simulink library "FoldingMechanisms"  (R2017a)
settings: Solver=VariableStepAuto  StartTime=0.0  StopTime=10.0  RelTol=1e-3
undefined symbols (not defined in the file or in its folder): X, Y, Z
libraries: sm_lib x70, FoldingMechanisms x62, nesl_utility x7
(part 3 of 4)

== system FoldingMechanisms/Vertices/5-Foldlines Vertices ==
  5-Foldlines : Subsystem  mask{angspec=zeros(5,1), angval=zeros(5,1)}
      mask prompts: angspec "Specify initial angles [nx1] (1/0)"; angval "Initial angles [nx1]"
      mask DialogControl DescTextVar Prompt: 5-Foldlines Vertex
      mask DialogControl Control2 Prompt: Here you can define initial values for foldlines, i.e. the configuration (valley/mountain fold or elbow up/elbow down or +1/-1). Thereby, you can define an angle and simulink will try to use that as the inital pose. Note, contradicting specification may lead to unexpected results. Please provide a vector with the size of the number of foldlines. First, provide an vector containing 0 or 1 to specifiy whether you want to use the initial value or not. Then, specify the initial angles.
      mask Display:
      | %This does not require changes,
      | %when the number of foldlines is changed.
      | n_myfoldlines=5;
      | 
      | FoldChars={'A','B','C','D','E','F','G','H','I','J','K','L','M','N'};
      | M=[0.5;0.5];
      | %Draw point in the middle
      | theta = 0 : 0.01 : 2*pi;
      | patch([M(1)+0.03*cos(theta)], [M(2)+0.03*sin(theta)], [0.8 0 0]);
      | %Draw n foldlines
      | 
      | gap=0.05;
      | chargap=0.06;
      | textboxcorrection=[0.03;-0.003];
      | R=0.35;
      | phi=linspace(90,90-360,n_myfoldlines+1);
      | for idx=1:n_myfoldlines
      |     cl=[0 0 0];
      |     %Print blue, if angspec is defined
      |     if angspec(idx)
      |        cl=[0 0 0.8];
      |     end
      |     %if actfoldlines(idx)
      |     %    cl=[0.8 0 0];
      |     %end
      |     startpos=M+gap*[cosd(phi(idx));sind(phi(idx))];
      |     endpos=startpos+R*[cosd(phi(idx));sind(phi(idx))];
      |     textposline=(startpos+endpos)/2;
      |     textpos1=textposline+chargap*[cosd(phi(idx)+90);sind(phi(idx)+90)]-textboxcorrection;
      |     textpos2=textposline+chargap*[cosd(phi(idx)-90);sind(phi(idx)-90)]-textboxcorrection;
      |     patch([startpos(1);endpos(1)],[startpos(2);endpos(2)],cl);
      |     text(textpos1(1),textpos1(2),[FoldChars{idx},'.',num2str(idx)]);
      |     if idx<n_myfoldlines
      |         text(textpos2(1),textpos2(2),[FoldChars{idx+1},'.',num2str(idx)]);
      |     else
      |         text(textpos2(1),textpos2(2),[FoldChars{1},'.',num2str(idx)]);
      |     end
      | end
  5-Foldlines-MotionInput : Subsystem  mask{angspec=zeros(5,1), angval=zeros(5,1), actdrive1=off, actdrive2=off, actdrive3=off, actdrive4=off, actdrive5=off}
      mask prompts: angspec "Specify initial angles [nx1] (1/0)"; angval "Initial angles [nx1]"; actdrive1 "Actuate Foldline1"; actdrive2 "Actuate Foldline2"; actdrive3 "Actuate Foldline3"; actdrive4 "Actuate Foldline4"; actdrive5 "Actuate Foldline5"
      mask init:
      | %Please provide number of foldlines here
      | n_myfoldlines=5;
      | 
      | n_actuation=0;
      | inputselector=ones(n_myfoldlines,1);
      | for idx=1:n_myfoldlines
      |     if eval(['actdrive',num2str(idx)])
      |         n_actuation=n_actuation+1;
      |         inputselector(idx)=n_actuation;
      |     end 
      | end
      mask TypeOptions actdrive1: Foldline1/actdrive
      mask TypeOptions actdrive2: Foldline2/actdrive
      mask TypeOptions actdrive3: Foldline3/actdrive
      mask TypeOptions actdrive4: Foldline4/actdrive
      mask TypeOptions actdrive5: Foldline5/actdrive
      mask DialogControl DescTextVar Prompt: 5-Foldlines Vertex with motion input
      mask DialogControl Control2 Prompt: Here you can define initial values for foldlines, i.e. the configuration (valley/mountain fold or elbow up/elbow down or +1/-1). Thereby, you can define an angle and simulink will try to use that as the inital pose. Note, contradicting specification may lead to unexpected results. Please provide a vector with the size of the number of foldlines. First, provide an vector containing 0 or 1 to specifiy whether you want to use the initial value or not. Then, specify the initial angles.
      mask Display:
      | %Please provide number of foldlines here
      | n_myfoldlines=5;
      | 
      | %This does not require changes
      | n_actuation=0;
      | FoldChars={'A','B','C','D','E','F','G','H','I','J','K','L','M','N'};
      | 
      | M=[0.5;0.5];
      | %Draw point in the middle
      | theta = 0 : 0.01 : 2*pi;
      | patch([M(1)+0.03*cos(theta)], [M(2)+0.03*sin(theta)], [0.8 0 0]);
      | %Draw n foldlines
      | 
      | gap=0.05;
      | chargap=0.06;
      | textboxcorrection=[0.03;-0.003];
      | R=0.35;
      | phi=linspace(90,90-360,n_myfoldlines+1);
      | for idx=1:n_myfoldlines
      |     cl=[0 0 0];
      |     if eval(['actdrive',num2str(idx)])
      |         cl=[0.8 0 0];
      |         n_actuation=n_actuation+1;
      |     end
      |     startpos=M+gap*[cosd(phi(idx));sind(phi(idx))];
      |     endpos=startpos+R*[cosd(phi(idx));sind(phi(idx))];
      |     textposline=(startpos+endpos)/2;
      |     textpos1=textposline+chargap*[cosd(phi(idx)+90);sind(phi(idx)+90)]-textboxcorrection;
      |     textpos2=textposline+chargap*[cosd(phi(idx)-90);sind(phi(idx)-90)]-textboxcorrection;
      |     patch([startpos(1);endpos(1)],[startpos(2);endpos(2)],cl);
      |     text(textpos1(1),textpos1(2),[FoldChars{idx},'.',num2str(idx)]);
      |     if idx<n_myfoldlines
      |         text(textpos2(1),textpos2(2),[FoldChars{idx+1},'.',num2str(idx)]);
      |     else
      |         text(textpos2(1),textpos2(2),[FoldChars{1},'.',num2str(idx)]);
      |     end
      | end
      | 
      | text(0.75,0.1,['F=',num2str(n_myfoldlines-3-n_actuation)]);

== system FoldingMechanisms/Vertices/6-Foldlines Vertices ==
  6-Foldlines : Subsystem  mask{angspec=zeros(6,1), angval=zeros(6,1)}
      mask prompts: angspec "Specify initial angles [nx1] (1/0)"; angval "Initial angles [nx1]"
      mask DialogControl DescTextVar Prompt: 6-Foldlines Vertex
      mask DialogControl Control2 Prompt: Here you can define initial values for foldlines, i.e. the configuration (valley/mountain fold or elbow up/elbow down or +1/-1). Thereby, you can define an angle and simulink will try to use that as the inital pose. Note, contradicting specification may lead to unexpected results. Please provide a vector with the size of the number of foldlines. First, provide an vector containing 0 or 1 to specifiy whether you want to use the initial value or not. Then, specify the initial angles.
      mask Display:
      | %This does not require changes,
      | %when the number of foldlines is changed.
      | n_myfoldlines=6;
      | 
      | FoldChars={'A','B','C','D','E','F','G','H','I','J','K','L','M','N'};
      | M=[0.5;0.5];
      | %Draw point in the middle
      | theta = 0 : 0.01 : 2*pi;
      | patch([M(1)+0.03*cos(theta)], [M(2)+0.03*sin(theta)], [0.8 0 0]);
      | %Draw n foldlines
      | 
      | gap=0.05;
      | chargap=0.06;
      | textboxcorrection=[0.03;-0.003];
      | R=0.35;
      | phi=linspace(90,90-360,n_myfoldlines+1);
      | for idx=1:n_myfoldlines
      |     cl=[0 0 0];
      |     %Print blue, if angspec is defined
      |     if angspec(idx)
      |        cl=[0 0 0.8];
      |     end
      |     %if actfoldlines(idx)
      |     %    cl=[0.8 0 0];
      |     %end
      |     startpos=M+gap*[cosd(phi(idx));sind(phi(idx))];
      |     endpos=startpos+R*[cosd(phi(idx));sind(phi(idx))];
      |     textposline=(startpos+endpos)/2;
      |     textpos1=textposline+chargap*[cosd(phi(idx)+90);sind(phi(idx)+90)]-textboxcorrection;
      |     textpos2=textposline+chargap*[cosd(phi(idx)-90);sind(phi(idx)-90)]-textboxcorrection;
      |     patch([startpos(1);endpos(1)],[startpos(2);endpos(2)],cl);
      |     text(textpos1(1),textpos1(2),[FoldChars{idx},'.',num2str(idx)]);
      |     if idx<n_myfoldlines
      |         text(textpos2(1),textpos2(2),[FoldChars{idx+1},'.',num2str(idx)]);
      |     else
      |         text(textpos2(1),textpos2(2),[FoldChars{1},'.',num2str(idx)]);
      |     end
      | end
  6-Foldlines-MotionInput : Subsystem  mask{angspec=zeros(6,1), angval=zeros(6,1), actdrive1=off, actdrive2=off, actdrive3=off, actdrive4=off, actdrive5=off, actdrive6=off}
      mask prompts: angspec "Specify initial angles [nx1] (1/0)"; angval "Initial angles [nx1]"; actdrive1 "Actuate Foldline1"; actdrive2 "Actuate Foldline2"; actdrive3 "Actuate Foldline3"; actdrive4 "Actuate Foldline4"; actdrive5 "Actuate Foldline5"; actdrive6 "Actuate Foldline6"
      mask init:
      | %Please provide number of foldlines here
      | n_myfoldlines=6;
      | 
      | n_actuation=0;
      | inputselector=ones(n_myfoldlines,1);
      | for idx=1:n_myfoldlines
      |      %Force run of initization commands
      |     eval(['actdrive',num2str(idx),'=~actdrive',num2str(idx),';']);
      |     eval(['actdrive',num2str(idx),'=~actdrive',num2str(idx),';']);
      |     if eval(['actdrive',num2str(idx)])
      |         n_actuation=n_actuation+1;
      |         inputselector(idx)=n_actuation;
      |     end 
      | end
      mask TypeOptions actdrive1: Foldline1/actdrive
      mask TypeOptions actdrive2: Foldline2/actdrive
      mask TypeOptions actdrive3: Foldline3/actdrive
      mask TypeOptions actdrive4: Foldline4/actdrive
      mask TypeOptions actdrive5: Foldline5/actdrive
      mask TypeOptions actdrive6: Foldline6/actdrive
      mask DialogControl DescTextVar Prompt: 6-Foldlines Vertex with motion input
      mask DialogControl Control2 Prompt: Here you can define initial values for foldlines, i.e. the configuration (valley/mountain fold or elbow up/elbow down or +1/-1). Thereby, you can define an angle and simulink will try to use that as the inital pose. Note, contradicting specification may lead to unexpected results. Please provide a vector with the size of the number of foldlines. First, provide an vector containing 0 or 1 to specifiy whether you want to use the initial value or not. Then, specify the initial angles.
      mask Display:
      | %Please provide number of foldlines here
      | n_myfoldlines=6;
      | 
      | %This does not require changes
      | n_actuation=0;
      | FoldChars={'A','B','C','D','E','F','G','H','I','J','K','L','M','N'};
      | 
      | M=[0.5;0.5];
      | %Draw point in the middle
      | theta = 0 : 0.01 : 2*pi;
      | patch([M(1)+0.03*cos(theta)], [M(2)+0.03*sin(theta)], [0.8 0 0]);
      | %Draw n foldlines
      | 
      | gap=0.05;
      | chargap=0.06;
      | textboxcorrection=[0.03;-0.003];
      | R=0.35;
      | phi=linspace(90,90-360,n_myfoldlines+1);
      | for idx=1:n_myfoldlines
      |     cl=[0 0 0];
      |     if eval(['actdrive',num2str(idx)])
      |         cl=[0.8 0 0];
      |         n_actuation=n_actuation+1;
      |     end
      |     startpos=M+gap*[cosd(phi(idx));sind(phi(idx))];
      |     endpos=startpos+R*[cosd(phi(idx));sind(phi(idx))];
      |     textposline=(startpos+endpos)/2;
      |     textpos1=textposline+chargap*[cosd(phi(idx)+90);sind(phi(idx)+90)]-textboxcorrection;
      |     textpos2=textposline+chargap*[cosd(phi(idx)-90);sind(phi(idx)-90)]-textboxcorrection;
      |     patch([startpos(1);endpos(1)],[startpos(2);endpos(2)],cl);
      |     text(textpos1(1),textpos1(2),[FoldChars{idx},'.',num2str(idx)]);
      |     if idx<n_myfoldlines
      |         text(textpos2(1),textpos2(2),[FoldChars{idx+1},'.',num2str(idx)]);
      |     else
      |         text(textpos2(1),textpos2(2),[FoldChars{1},'.',num2str(idx)]);
      |     end
      | end
      | 
      | text(0.75,0.1,['F=',num2str(n_myfoldlines-3-n_actuation)]);

== system FoldingMechanisms/Vertices/7-Foldlines Vertices ==
  7-Foldlines : Subsystem  mask{angspec=zeros(7,1), angval=zeros(7,1)}
      mask prompts: angspec "Specify initial angles [nx1] (1/0)"; angval "Initial angles [nx1]"
      mask DialogControl DescTextVar Prompt: 7-Foldlines Vertex
      mask DialogControl Control2 Prompt: Here you can define initial values for foldlines, i.e. the configuration (valley/mountain fold or elbow up/elbow down or +1/-1). Thereby, you can define an angle and simulink will try to use that as the inital pose. Note, contradicting specification may lead to unexpected results. Please provide a vector with the size of the number of foldlines. First, provide an vector containing 0 or 1 to specifiy whether you want to use the initial value or not. Then, specify the initial angles.
      mask Display:
      | %This does not require changes,
      | %when the number of foldlines is changed.
      | n_myfoldlines=7;
      | 
      | FoldChars={'A','B','C','D','E','F','G','H','I','J','K','L','M','N'};
      | M=[0.5;0.5];
      | %Draw point in the middle
      | theta = 0 : 0.01 : 2*pi;
      | patch([M(1)+0.03*cos(theta)], [M(2)+0.03*sin(theta)], [0.8 0 0]);
      | %Draw n foldlines
      | 
      | gap=0.05;
      | chargap=0.06;
      | textboxcorrection=[0.03;-0.003];
      | R=0.35;
      | phi=linspace(90,90-360,n_myfoldlines+1);
      | for idx=1:n_myfoldlines
      |     cl=[0 0 0];
      |     %Print blue, if angspec is defined
      |     if angspec(idx)
      |        cl=[0 0 0.8];
      |     end
      |     %if actfoldlines(idx)
      |     %    cl=[0.8 0 0];
      |     %end
      |      startpos=M+gap*[cosd(phi(idx));sind(phi(idx))];
      |     endpos=startpos+R*[cosd(phi(idx));sind(phi(idx))];
      |     textposline=startpos+R/1.3*[cosd(phi(idx));sind(phi(idx))];
      |     textpos1=textposline+chargap*[cosd(phi(idx)+90);sind(phi(idx)+90)]-textboxcorrection;
      |     textpos2=textposline+chargap*[cosd(phi(idx)-90);sind(phi(idx)-90)]-textboxcorrection;
      |     patch([startpos(1);endpos(1)],[startpos(2);endpos(2)],cl);
      |     text(textpos1(1),textpos1(2),[FoldChars{idx},'.',num2str(idx)]);
      |     if idx<n_myfoldlines
      |         text(textpos2(1),textpos2(2),[FoldChars{idx+1},'.',num2str(idx)]);
      |     else
      |         text(textpos2(1),textpos2(2),[FoldChars{1},'.',num2str(idx)]);
      |     end
      | end
  7-Foldlines-MotionInput : Subsystem  mask{angspec=zeros(7,1), angval=zeros(7,1), actdrive1=off, actdrive2=off, actdrive3=off, actdrive4=off, actdrive5=off, actdrive6=off, actdrive7=off}
      mask prompts: angspec "Specify initial angles [nx1] (1/0)"; angval "Initial angles [nx1]"; actdrive1 "Actuate Foldline1"; actdrive2 "Actuate Foldline2"; actdrive3 "Actuate Foldline3"; actdrive4 "Actuate Foldline4"; actdrive5 "Actuate Foldline5"; actdrive6 "Actuate Foldline6"; actdrive7 "Actuate Foldline7"
      mask init:
      | %Please provide number of foldlines here
      | n_myfoldlines=7;
      | 
      | n_actuation=0;
      | inputselector=ones(n_myfoldlines,1);
      | for idx=1:n_myfoldlines
      |      %Force run of initization commands
      |     eval(['actdrive',num2str(idx),'=~actdrive',num2str(idx),';']);
      |     eval(['actdrive',num2str(idx),'=~actdrive',num2str(idx),';']);
      |     if eval(['actdrive',num2str(idx)])
      |         n_actuation=n_actuation+1;
      |         inputselector(idx)=n_actuation;
      |     end 
      | end
      mask TypeOptions actdrive1: Foldline1/actdrive
      mask TypeOptions actdrive2: Foldline2/actdrive
      mask TypeOptions actdrive3: Foldline3/actdrive
      mask TypeOptions actdrive4: Foldline4/actdrive
      mask TypeOptions actdrive5: Foldline5/actdrive
      mask TypeOptions actdrive6: Foldline6/actdrive
      mask TypeOptions actdrive7: Foldline7/actdrive
      mask DialogControl DescTextVar Prompt: 7-Foldlines Vertex with motion input
      mask DialogControl Control2 Prompt: Here you can define initial values for foldlines, i.e. the configuration (valley/mountain fold or elbow up/elbow down or +1/-1). Thereby, you can define an angle and simulink will try to use that as the inital pose. Note, contradicting specification may lead to unexpected results. Please provide a vector with the size of the number of foldlines. First, provide an vector containing 0 or 1 to specifiy whether you want to use the initial value or not. Then, specify the initial angles.
      mask Display:
      | %Please provide number of foldlines here
      | n_myfoldlines=7;
      | 
      | %This does not require changes
      | n_actuation=0;
      | FoldChars={'A','B','C','D','E','F','G','H','I','J','K','L','M','N'};
      | 
      | M=[0.5;0.5];
      | %Draw point in the middle
      | theta = 0 : 0.01 : 2*pi;
      | patch([M(1)+0.03*cos(theta)], [M(2)+0.03*sin(theta)], [0.8 0 0]);
      | %Draw n foldlines
      | 
      | gap=0.05;
      | chargap=0.06;
      | textboxcorrection=[0.03;-0.003];
      | R=0.35;
      | phi=linspace(90,90-360,n_myfoldlines+1);
      | for idx=1:n_myfoldlines
      |     cl=[0 0 0];
      |     if eval(['actdrive',num2str(idx)])
      |         cl=[0.8 0 0];
      |         n_actuation=n_actuation+1;
      |     end
      |     startpos=M+gap*[cosd(phi(idx));sind(phi(idx))];
      |     endpos=startpos+R*[cosd(phi(idx));sind(phi(idx))];
      |     textposline=startpos+R/1.3*[cosd(phi(idx));sind(phi(idx))];
      |     textpos1=textposline+chargap*[cosd(phi(idx)+90);sind(phi(idx)+90)]-textboxcorrection;
      |     textpos2=textposline+chargap*[cosd(phi(idx)-90);sind(phi(idx)-90)]-textboxcorrection;
      |     patch([startpos(1);endpos(1)],[startpos(2);endpos(2)],cl);
      |     text(textpos1(1),textpos1(2),[FoldChars{idx},'.',num2str(idx)]);
      |     if idx<n_myfoldlines
      |         text(textpos2(1),textpos2(2),[FoldChars{idx+1},'.',num2str(idx)]);
      |     else
      |         text(textpos2(1),textpos2(2),[FoldChars{1},'.',num2str(idx)]);
      |     end
      | end
      | 
      | text(0.75,0.1,['F=',num2str(n_myfoldlines-3-n_actuation)]);

== system FoldingMechanisms/Vertices/8-Foldlines Vertices ==
  8-Foldlines : Subsystem  mask{angspec=zeros(8,1), angval=zeros(8,1)}
      mask prompts: angspec "Specify initial angles [nx1] (1/0)"; angval "Initial angles [nx1]"
      mask DialogControl DescTextVar Prompt: 8-Foldlines Vertex
      mask DialogControl Control2 Prompt: Here you can define initial values for foldlines, i.e. the configuration (valley/mountain fold or elbow up/elbow down or +1/-1). Thereby, you can define an angle and simulink will try to use that as the inital pose. Note, contradicting specification may lead to unexpected results. Please provide a vector with the size of the number of foldlines. First, provide an vector containing 0 or 1 to specifiy whether you want to use the initial value or not. Then, specify the initial angles.
      mask Display:
      | %This does not require changes,
      | %when the number of foldlines is changed.
      | n_myfoldlines=8;
      | 
      | FoldChars={'A','B','C','D','E','F','G','H','I','J','K','L','M','N'};
      | M=[0.5;0.5];
      | %Draw point in the middle
      | theta = 0 : 0.01 : 2*pi;
      | patch([M(1)+0.03*cos(theta)], [M(2)+0.03*sin(theta)], [0.8 0 0]);
      | %Draw n foldlines
      | 
      | gap=0.05;
      | chargap=0.06;
      | textboxcorrection=[0.03;-0.003];
      | R=0.35;
      | phi=linspace(90,90-360,n_myfoldlines+1);
      | for idx=1:n_myfoldlines
      |     cl=[0 0 0];
      |     %Print blue, if angspec is defined
      |     if angspec(idx)
      |        cl=[0 0 0.8];
      |     end
      |     %if actfoldlines(idx)
      |     %    cl=[0.8 0 0];
      |     %end
      |      startpos=M+gap*[cosd(phi(idx));sind(phi(idx))];
      |     endpos=startpos+R*[cosd(phi(idx));sind(phi(idx))];
      |     textposline=startpos+R/1.25*[cosd(phi(idx));sind(phi(idx))];
      |     textpos1=textposline+chargap*[cosd(phi(idx)+90);sind(phi(idx)+90)]-textboxcorrection;
      |     textpos2=textposline+chargap*[cosd(phi(idx)-90);sind(phi(idx)-90)]-textboxcorrection;
      |     patch([startpos(1);endpos(1)],[startpos(2);endpos(2)],cl);
      |     text(textpos1(1),textpos1(2),[FoldChars{idx},'.',num2str(idx)]);
      |     if idx<n_myfoldlines
      |         text(textpos2(1),textpos2(2),[FoldChars{idx+1},'.',num2str(idx)]);
      |     else
      |         text(textpos2(1),textpos2(2),[FoldChars{1},'.',num2str(idx)]);
      |     end
      | end
  8-Foldlines-MotionInput : Subsystem  mask{angspec=zeros(8,1), angval=zeros(8,1), actdrive1=off, actdrive2=off, actdrive3=off, actdrive4=off, actdrive5=off, actdrive6=off, actdrive7=off, actdrive8=off}
      mask prompts: angspec "Specify initial angles [nx1] (1/0)"; angval "Initial angles [nx1]"; actdrive1 "Actuate Foldline1"; actdrive2 "Actuate Foldline2"; actdrive3 "Actuate Foldline3"; actdrive4 "Actuate Foldline4"; actdrive5 "Actuate Foldline5"; actdrive6 "Actuate Foldline6"; actdrive7 "Actuate Foldline7"; actdrive8 "Actuate Foldline8"
      mask init:
      | %Please provide number of foldlines here
      | n_myfoldlines=8;
      | 
      | n_actuation=0;
      | inputselector=ones(n_myfoldlines,1);
      | for idx=1:n_myfoldlines
      |      %Force run of initization commands
      |     eval(['actdrive',num2str(idx),'=~actdrive',num2str(idx),';']);
      |     eval(['actdrive',num2str(idx),'=~actdrive',num2str(idx),';']);
      |     if eval(['actdrive',num2str(idx)])
      |         n_actuation=n_actuation+1;
      |         inputselector(idx)=n_actuation;
      |     end 
      | end
      mask TypeOptions actdrive1: Foldline1/actdrive
      mask TypeOptions actdrive2: Foldline2/actdrive
      mask TypeOptions actdrive3: Foldline3/actdrive
      mask TypeOptions actdrive4: Foldline4/actdrive
      mask TypeOptions actdrive5: Foldline5/actdrive
      mask TypeOptions actdrive6: Foldline6/actdrive
      mask TypeOptions actdrive7: Foldline7/actdrive
      mask TypeOptions actdrive8: Foldline8/actdrive
      mask DialogControl DescTextVar Prompt: 8-Foldlines Vertex with motion input
      mask DialogControl Control2 Prompt: Here you can define initial values for foldlines, i.e. the configuration (valley/mountain fold or elbow up/elbow down or +1/-1). Thereby, you can define an angle and simulink will try to use that as the inital pose. Note, contradicting specification may lead to unexpected results. Please provide a vector with the size of the number of foldlines. First, provide an vector containing 0 or 1 to specifiy whether you want to use the initial value or not. Then, specify the initial angles.
      mask Display:
      | %Please provide number of foldlines here
      | n_myfoldlines=8;
      | 
      | %This does not require changes
      | n_actuation=0;
      | FoldChars={'A','B','C','D','E','F','G','H','I','J','K','L','M','N'};
      | 
      | M=[0.5;0.5];
      | %Draw point in the middle
      | theta = 0 : 0.01 : 2*pi;
      | patch([M(1)+0.03*cos(theta)], [M(2)+0.03*sin(theta)], [0.8 0 0]);
      | %Draw n foldlines
      | 
      | gap=0.05;
      | chargap=0.06;
      | textboxcorrection=[0.03;-0.003];
      | R=0.35;
      | phi=linspace(90,90-360,n_myfoldlines+1);
      | for idx=1:n_myfoldlines
      |     cl=[0 0 0];
      |     if eval(['actdrive',num2str(idx)])
      |         cl=[0.8 0 0];
      |         n_actuation=n_actuation+1;
      |     end
      |     startpos=M+gap*[cosd(phi(idx));sind(phi(idx))];
      |     endpos=startpos+R*[cosd(phi(idx));sind(phi(idx))];
      |     textposline=startpos+R/1.3*[cosd(phi(idx));sind(phi(idx))];
      |     textpos1=textposline+chargap*[cosd(phi(idx)+90);sind(phi(idx)+90)]-textboxcorrection;
      |     textpos2=textposline+chargap*[cosd(phi(idx)-90);sind(phi(idx)-90)]-textboxcorrection;
      |     patch([startpos(1);endpos(1)],[startpos(2);endpos(2)],cl);
      |     text(textpos1(1),textpos1(2),[FoldChars{idx},'.',num2str(idx)]);
      |     if idx<n_myfoldlines
      |         text(textpos2(1),textpos2(2),[FoldChars{idx+1},'.',num2str(idx)]);
      |     else
      |         text(textpos2(1),textpos2(2),[FoldChars{1},'.',num2str(idx)]);
      |     end
      | end
      | 
      | text(0.75,0.1,['F=',num2str(n_myfoldlines-3-n_actuation)]);

== system FoldingMechanisms/Vertices/Subelements ==
  Single Driven Foldline : Subsystem
      mask DialogControl DescGroupVar Prompt: Single Driven Foldline
      mask DialogControl DescTextVar Prompt: This block provides a single driven Foldline.
      mask Display: patch([0.5 0.5],[0.2 0.8],[0.8 0 0]);
  Single Foldline : Subsystem  mask{angleAB=0, specAngleAB=0}
      mask prompts: angleAB "Angle [°]"; specAngleAB "Specify Configuration [true/false]"
      mask init:
      | %Initialize
      | if (specAngleAB==true)
      |     set_param([gcb,'/Foldline'], 'PositionTargetSpecify','on');
      | else
      |     set_param([gcb,'/Foldline'], 'PositionTargetSpecify','off');
      | end
      mask DialogControl DescTextVar Prompt: This block provides the definition of a single Foldline with the possibility to specify the configuration
      mask Display: plot([0.5 0.5],[0.2 0.8]);
  Variant Foldline : Subsystem  LoadFcn=|  Variant=on  OverrideUsingVariant=Foldline  mask{angleAB=0, specAngleAB=0, actdrive=off, chooseVariant=Foldline}
      | actdrive = get_param(gcb,'actdrive');
      | if strcmp(actdrive,'on')
      |     set_param(gcb,'chooseVariant','Drive');
      | else
      |     set_param(gcb,'chooseVariant','Foldline');
      | end
      mask prompts: angleAB "Angle [°]"; specAngleAB "Specify Configuration [true/false]"; actdrive "Driven"; chooseVariant "Simulink:blkprm_prompts:OverrideUsingVariant"
      mask init:
      | actdrive = get_param(gcb,'actdrive');
      | if strcmp(actdrive,'on')
      |     set_param(gcb,'chooseVariant','Drive');
      | else
      |     set_param(gcb,'chooseVariant','Foldline');
      | end
      mask Callback actdrive:
      | actdrive = get_param(gcb,'actdrive');
      | if strcmp(actdrive,'on')
      |     set_param(gcb,'chooseVariant','Drive');
      | else
      |     set_param(gcb,'chooseVariant','Foldline');
      | end
      mask TypeOptions chooseVariant: OverrideUsingVariant
      mask DialogControl DescTextVar Prompt: This is a variant Foldline. You can choose, whether this Foldline is actuated. If actuated, Foldline specifications will be ignored. If not actuated, the drive function will be ignored.
      mask Display:
      | if strcmp(actdrive,'on');
      |     patch([0.5 0.5],[0.2 0.8],[0.8 0 0]);
      | else
      |     patch([0.5 0.5],[0.2 0.8],[0 0 0]);
      | end

== system FoldingMechanisms/Vertices/4-Foldlines Vertices/4-Foldlines ==
  Bus Creator4 : BusCreator  Inputs=4
  Foldline AB : FoldingMechanisms/Vertices/Subelements/Single Foldline  angleAB=angval(1)  specAngleAB=angspec(1)
      settings: SourceProductName=FoldingMechanisms
  Foldline AD : FoldingMechanisms/Vertices/Subelements/Single Foldline  angleAB=angval(4)  specAngleAB=angspec(4)
      settings: SourceProductName=FoldingMechanisms
  Foldline CB : FoldingMechanisms/Vertices/Subelements/Single Foldline  angleAB=angval(2)  specAngleAB=angspec(2)
      settings: SourceProductName=FoldingMechanisms
  Foldline CD : FoldingMechanisms/Vertices/Subelements/Single Foldline  angleAB=angval(3)  specAngleAB=angspec(2)
      settings: SourceProductName=FoldingMechanisms
  A1 : PMIOPort  Port=1  Side=Left
  A4 : PMIOPort  Port=2  Side=Left
  D4 : PMIOPort  Port=3  Side=Left
  D3 : PMIOPort  Port=4  Side=Left
  B1 : PMIOPort  Port=5  Side=Right
  B2 : PMIOPort  Port=6  Side=Right
  C2 : PMIOPort  Port=7  Side=Right
  C3 : PMIOPort  Port=8  Side=Right
  Out Bus Element : Outport  PortName=OutBus  Element=Sensing
  wires:
  Bus Creator4/1 -> Out Bus Element/1
  Foldline AB/1 -> Bus Creator4/1
  Foldline AD/1 -> Bus Creator4/4
  Foldline CD/1 -> Bus Creator4/3
  Foldline CB/1 -> Bus Creator4/2
  connections:
  Foldline CB/RConn1 -- B2/RConn1
  Foldline AB/LConn1 -- A1/RConn1
  Foldline AB/RConn1 -- B1/RConn1
  D4/RConn1 -- Foldline AD/LConn1
  A4/RConn1 -- Foldline AD/RConn1
  Foldline CD/LConn1 -- D3/RConn1
  Foldline CD/RConn1 -- C3/RConn1
  C2/RConn1 -- Foldline CB/LConn1

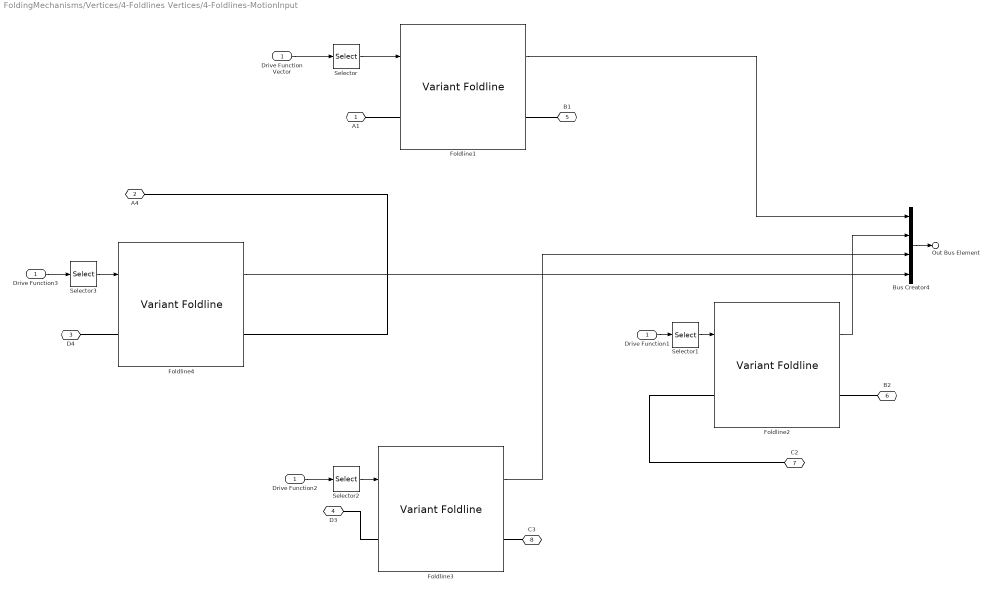
== system FoldingMechanisms/Vertices/4-Foldlines Vertices/4-Foldlines-MotionInput ==
  Drive Function Vector : Inport
  Bus Creator4 : BusCreator  Inputs=4
  Drive Function1 : InportShadow
  Drive Function2 : InportShadow
  Drive Function3 : InportShadow
  Foldline1 : FoldingMechanisms/Vertices/Subelements/Variant Foldline  angleAB=angval(1)  specAngleAB=angspec(1)  actdrive=off  chooseVariant=Foldline
      settings: SourceProductName=FoldingMechanisms
  Foldline2 : FoldingMechanisms/Vertices/Subelements/Variant Foldline  angleAB=angval(2)  specAngleAB=angspec(2)  actdrive=off  chooseVariant=Foldline
      settings: SourceProductName=FoldingMechanisms
  Foldline3 : FoldingMechanisms/Vertices/Subelements/Variant Foldline  angleAB=angval(3)  specAngleAB=angspec(3)  actdrive=off  chooseVariant=Foldline
      settings: SourceProductName=FoldingMechanisms
  Foldline4 : FoldingMechanisms/Vertices/Subelements/Variant Foldline  angleAB=angval(4)  specAngleAB=angspec(4)  actdrive=off  chooseVariant=Foldline
      settings: SourceProductName=FoldingMechanisms
  Selector : Selector  InputPortWidth=max(n_actuation,1)  IndexOptions=Index vector (dialog)  Indices=inputselector(1)  OutputSizes=1
  Selector1 : Selector  InputPortWidth=max(n_actuation,1)  IndexOptions=Index vector (dialog)  Indices=inputselector(2)  OutputSizes=1
  Selector2 : Selector  InputPortWidth=max(n_actuation,1)  IndexOptions=Index vector (dialog)  Indices=inputselector(3)  OutputSizes=1
  Selector3 : Selector  InputPortWidth=max(n_actuation,1)  IndexOptions=Index vector (dialog)  Indices=inputselector(4)  OutputSizes=1
  A1 : PMIOPort  Port=1  Side=Left
  A4 : PMIOPort  Port=2  Side=Left
  D4 : PMIOPort  Port=3  Side=Left
  D3 : PMIOPort  Port=4  Side=Left
  B1 : PMIOPort  Port=5  Side=Right
  B2 : PMIOPort  Port=6  Side=Right
  C2 : PMIOPort  Port=7  Side=Right
  C3 : PMIOPort  Port=8  Side=Right
  Out Bus Element : Outport  PortName=OutBus  Element=Sensing
  wires:
  Bus Creator4/1 -> Out Bus Element/1
  Drive Function Vector/1 -> Selector/1
  Foldline1/1 -> Bus Creator4/1
  Foldline4/1 -> Bus Creator4/4
  Foldline3/1 -> Bus Creator4/3
  Foldline2/1 -> Bus Creator4/2
  Drive Function1/1 -> Selector1/1
  Drive Function2/1 -> Selector2/1
  Drive Function3/1 -> Selector3/1
  Selector/1 -> Foldline1/1
  Selector1/1 -> Foldline2/1
  Selector2/1 -> Foldline3/1
  Selector3/1 -> Foldline4/1
  connections:
  Foldline2/RConn1 -- B2/RConn1
  Foldline1/LConn1 -- A1/RConn1
  Foldline1/RConn1 -- B1/RConn1
  Foldline4/LConn1 -- D4/RConn1
  Foldline4/RConn1 -- A4/RConn1
  Foldline3/LConn1 -- D3/RConn1
  Foldline3/RConn1 -- C3/RConn1
  Foldline2/LConn1 -- C2/RConn1

== system FoldingMechanisms/Vertices/5-Foldlines Vertices/5-Foldlines ==
  Bus Creator4 : BusCreator  Inputs=5
  Foldline AB : FoldingMechanisms/Vertices/Subelements/Single Foldline  angleAB=angval(1)  specAngleAB=angspec(1)
      settings: SourceProductName=FoldingMechanisms
  Foldline AD : FoldingMechanisms/Vertices/Subelements/Single Foldline  angleAB=angval(4)  specAngleAB=angspec(4)
      settings: SourceProductName=FoldingMechanisms
  Foldline AD1 : FoldingMechanisms/Vertices/Subelements/Single Foldline  angleAB=angval(4)  specAngleAB=angspec(4)
      settings: SourceProductName=FoldingMechanisms
  Foldline CB : FoldingMechanisms/Vertices/Subelements/Single Foldline  angleAB=angval(2)  specAngleAB=angspec(2)
      settings: SourceProductName=FoldingMechanisms
  Foldline CD : FoldingMechanisms/Vertices/Subelements/Single Foldline  angleAB=angval(3)  specAngleAB=angspec(2)
      settings: SourceProductName=FoldingMechanisms
  A1 : PMIOPort  Port=1  Side=Left
  A5 : PMIOPort  Port=2  Side=Left
  E5 : PMIOPort  Port=3  Side=Left
  E4 : PMIOPort  Port=4  Side=Left
  D4 : PMIOPort  Port=5  Side=Left
  B1 : PMIOPort  Port=6  Side=Right
  B2 : PMIOPort  Port=7  Side=Right
  C2 : PMIOPort  Port=8  Side=Right
  C3 : PMIOPort  Port=9  Side=Right
  D3 : PMIOPort  Port=10  Side=Right
  Out Bus Element : Outport  PortName=OutBus  Element=Sensing
  wires:
  Bus Creator4/1 -> Out Bus Element/1
  Foldline AB/1 -> Bus Creator4/1
  Foldline AD/1 -> Bus Creator4/4
  Foldline CD/1 -> Bus Creator4/3
  Foldline CB/1 -> Bus Creator4/2
  Foldline AD1/1 -> Bus Creator4/5
  connections:
  Foldline CB/RConn1 -- B2/RConn1
  Foldline AB/LConn1 -- A1/RConn1
  Foldline AB/RConn1 -- B1/RConn1
  D4/RConn1 -- Foldline AD/LConn1
  E4/RConn1 -- Foldline AD/RConn1
  Foldline CD/LConn1 -- D3/RConn1
  Foldline CD/RConn1 -- C3/RConn1
  C2/RConn1 -- Foldline CB/LConn1
  A5/RConn1 -- Foldline AD1/RConn1
  E5/RConn1 -- Foldline AD1/LConn1

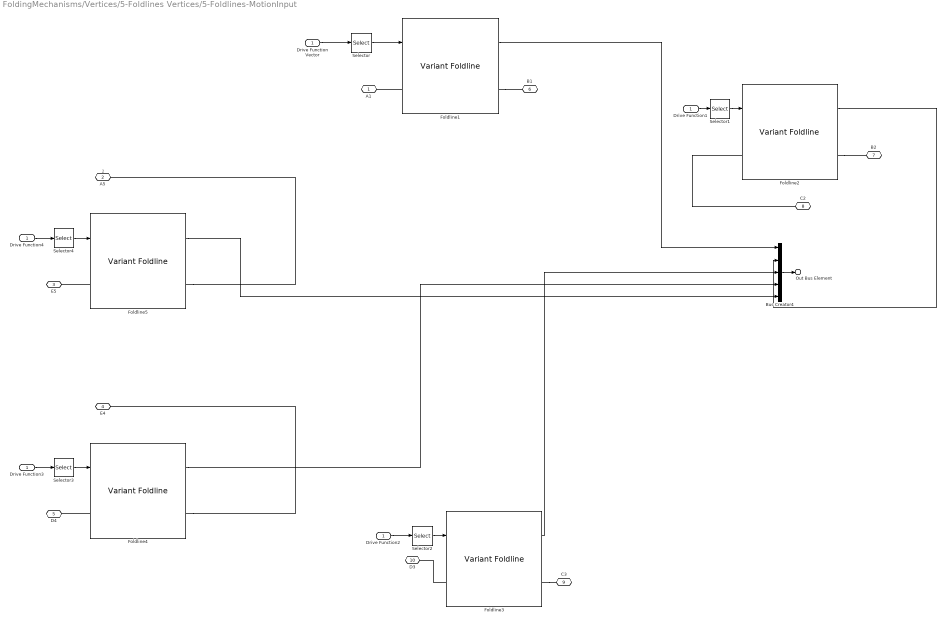
== system FoldingMechanisms/Vertices/5-Foldlines Vertices/5-Foldlines-MotionInput ==
  note: 2
  Drive Function Vector : Inport
  Bus Creator4 : BusCreator  Inputs=5
  Drive Function{1..4} (4 alike) : InportShadow
  Foldline1 : FoldingMechanisms/Vertices/Subelements/Variant Foldline  angleAB=angval(1)  specAngleAB=angspec(1)  actdrive=off  chooseVariant=Foldline
      settings: SourceProductName=FoldingMechanisms
  Foldline2 : FoldingMechanisms/Vertices/Subelements/Variant Foldline  angleAB=angval(2)  specAngleAB=angspec(2)  actdrive=off  chooseVariant=Foldline
      settings: SourceProductName=FoldingMechanisms
  Foldline3 : FoldingMechanisms/Vertices/Subelements/Variant Foldline  angleAB=angval(3)  specAngleAB=angspec(3)  actdrive=off  chooseVariant=Foldline
      settings: SourceProductName=FoldingMechanisms
  Foldline4 : FoldingMechanisms/Vertices/Subelements/Variant Foldline  angleAB=angval(4)  specAngleAB=angspec(4)  actdrive=off  chooseVariant=Foldline
      settings: SourceProductName=FoldingMechanisms
  Foldline5 : FoldingMechanisms/Vertices/Subelements/Variant Foldline  angleAB=angval(5)  specAngleAB=angspec(5)  actdrive=off  chooseVariant=Foldline
      settings: SourceProductName=FoldingMechanisms
  Selector : Selector  InputPortWidth=max(n_actuation,1)  IndexOptions=Index vector (dialog)  Indices=inputselector(1)  OutputSizes=1
  Selector1 : Selector  InputPortWidth=max(n_actuation,1)  IndexOptions=Index vector (dialog)  Indices=inputselector(2)  OutputSizes=1
  Selector2 : Selector  InputPortWidth=max(n_actuation,1)  IndexOptions=Index vector (dialog)  Indices=inputselector(3)  OutputSizes=1
  Selector3 : Selector  InputPortWidth=max(n_actuation,1)  IndexOptions=Index vector (dialog)  Indices=inputselector(4)  OutputSizes=1
  Selector4 : Selector  InputPortWidth=max(n_actuation,1)  IndexOptions=Index vector (dialog)  Indices=inputselector(5)  OutputSizes=1
  A1 : PMIOPort  Port=1  Side=Left
  A5 : PMIOPort  Port=2  Side=Left
  E5 : PMIOPort  Port=3  Side=Left
  E4 : PMIOPort  Port=4  Side=Left
  D4 : PMIOPort  Port=5  Side=Left
  B1 : PMIOPort  Port=6  Side=Right
  B2 : PMIOPort  Port=7  Side=Right
  C2 : PMIOPort  Port=8  Side=Right
  C3 : PMIOPort  Port=9  Side=Right
  D3 : PMIOPort  Port=10  Side=Right
  Out Bus Element : Outport  PortName=OutBus  Element=Sensing
  wires:
  Bus Creator4/1 -> Out Bus Element/1
  Drive Function Vector/1 -> Selector/1
  Foldline1/1 -> Bus Creator4/1
  Foldline4/1 -> Bus Creator4/4
  Foldline3/1 -> Bus Creator4/3
  Foldline2/1 -> Bus Creator4/2
  Drive Function1/1 -> Selector1/1
  Drive Function2/1 -> Selector2/1
  Drive Function3/1 -> Selector3/1
  Selector/1 -> Foldline1/1
  Selector1/1 -> Foldline2/1
  Selector2/1 -> Foldline3/1
  Selector3/1 -> Foldline4/1
  Drive Function4/1 -> Selector4/1
  Selector4/1 -> Foldline5/1
  Foldline5/1 -> Bus Creator4/5
  connections:
  Foldline2/RConn1 -- B2/RConn1
  Foldline1/LConn1 -- A1/RConn1
  Foldline1/RConn1 -- B1/RConn1
  Foldline4/LConn1 -- D4/RConn1
  Foldline4/RConn1 -- E4/RConn1
  Foldline3/LConn1 -- D3/RConn1
  Foldline3/RConn1 -- C3/RConn1
  Foldline2/LConn1 -- C2/RConn1
  Foldline5/LConn1 -- E5/RConn1
  Foldline5/RConn1 -- A5/RConn1

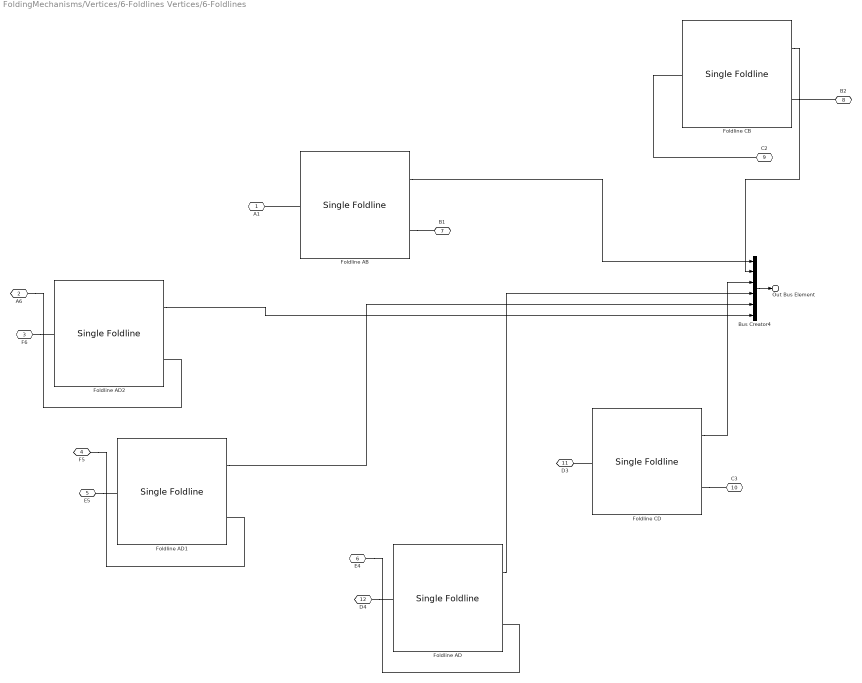
== system FoldingMechanisms/Vertices/6-Foldlines Vertices/6-Foldlines ==
  Bus Creator4 : BusCreator  Inputs=6
  Foldline AB : FoldingMechanisms/Vertices/Subelements/Single Foldline  angleAB=angval(1)  specAngleAB=angspec(1)
      settings: SourceProductName=FoldingMechanisms
  Foldline AD : FoldingMechanisms/Vertices/Subelements/Single Foldline  angleAB=angval(4)  specAngleAB=angspec(4)
      settings: SourceProductName=FoldingMechanisms
  Foldline AD1 : FoldingMechanisms/Vertices/Subelements/Single Foldline  angleAB=angval(4)  specAngleAB=angspec(4)
      settings: SourceProductName=FoldingMechanisms
  Foldline AD2 : FoldingMechanisms/Vertices/Subelements/Single Foldline  angleAB=angval(4)  specAngleAB=angspec(4)
      settings: SourceProductName=FoldingMechanisms
  Foldline CB : FoldingMechanisms/Vertices/Subelements/Single Foldline  angleAB=angval(2)  specAngleAB=angspec(2)
      settings: SourceProductName=FoldingMechanisms
  Foldline CD : FoldingMechanisms/Vertices/Subelements/Single Foldline  angleAB=angval(3)  specAngleAB=angspec(2)
      settings: SourceProductName=FoldingMechanisms
  A1 : PMIOPort  Port=1  Side=Left
  A6 : PMIOPort  Port=2  Side=Left
  F6 : PMIOPort  Port=3  Side=Left
  F5 : PMIOPort  Port=4  Side=Left
  E5 : PMIOPort  Port=5  Side=Left
  E4 : PMIOPort  Port=6  Side=Left
  B1 : PMIOPort  Port=7  Side=Right
  B2 : PMIOPort  Port=8  Side=Right
  C2 : PMIOPort  Port=9  Side=Right
  C3 : PMIOPort  Port=10  Side=Right
  D3 : PMIOPort  Port=11  Side=Right
  D4 : PMIOPort  Port=12  Side=Right
  Out Bus Element : Outport  PortName=OutBus  Element=Sensing
  wires:
  Bus Creator4/1 -> Out Bus Element/1
  Foldline AB/1 -> Bus Creator4/1
  Foldline AD/1 -> Bus Creator4/4
  Foldline CD/1 -> Bus Creator4/3
  Foldline CB/1 -> Bus Creator4/2
  Foldline AD1/1 -> Bus Creator4/5
  Foldline AD2/1 -> Bus Creator4/6
  connections:
  Foldline CB/RConn1 -- B2/RConn1
  Foldline AB/LConn1 -- A1/RConn1
  Foldline AB/RConn1 -- B1/RConn1
  D4/RConn1 -- Foldline AD/LConn1
  E4/RConn1 -- Foldline AD/RConn1
  Foldline CD/LConn1 -- D3/RConn1
  Foldline CD/RConn1 -- C3/RConn1
  C2/RConn1 -- Foldline CB/LConn1
  F5/RConn1 -- Foldline AD1/RConn1
  E5/RConn1 -- Foldline AD1/LConn1
  F6/RConn1 -- Foldline AD2/LConn1
  A6/RConn1 -- Foldline AD2/RConn1

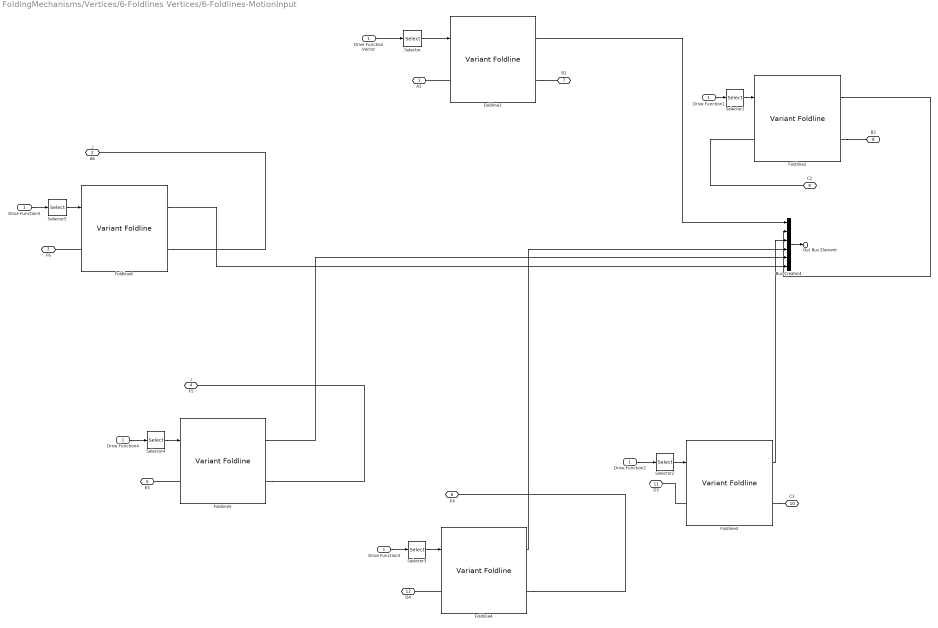
== system FoldingMechanisms/Vertices/6-Foldlines Vertices/6-Foldlines-MotionInput ==
  note: 2
  note: 2
  Drive Function Vector : Inport
  Bus Creator4 : BusCreator  Inputs=6
  Drive Function{1..5} (5 alike) : InportShadow
  Foldline1 : FoldingMechanisms/Vertices/Subelements/Variant Foldline  angleAB=angval(1)  specAngleAB=angspec(1)  actdrive=off  chooseVariant=Foldline
      settings: SourceProductName=FoldingMechanisms
  Foldline2 : FoldingMechanisms/Vertices/Subelements/Variant Foldline  angleAB=angval(2)  specAngleAB=angspec(2)  actdrive=off  chooseVariant=Foldline
      settings: SourceProductName=FoldingMechanisms
  Foldline3 : FoldingMechanisms/Vertices/Subelements/Variant Foldline  angleAB=angval(3)  specAngleAB=angspec(3)  actdrive=off  chooseVariant=Foldline
      settings: SourceProductName=FoldingMechanisms
  Foldline4 : FoldingMechanisms/Vertices/Subelements/Variant Foldline  angleAB=angval(4)  specAngleAB=angspec(4)  actdrive=off  chooseVariant=Foldline
      settings: SourceProductName=FoldingMechanisms
  Foldline5 : FoldingMechanisms/Vertices/Subelements/Variant Foldline  angleAB=angval(5)  specAngleAB=angspec(5)  actdrive=off  chooseVariant=Foldline
      settings: SourceProductName=FoldingMechanisms
  Foldline6 : FoldingMechanisms/Vertices/Subelements/Variant Foldline  angleAB=angval(6)  specAngleAB=angspec(6)  actdrive=off  chooseVariant=Foldline
      settings: SourceProductName=FoldingMechanisms
  Selector : Selector  InputPortWidth=max(n_actuation,1)  IndexOptions=Index vector (dialog)  Indices=inputselector(1)  OutputSizes=1
  Selector1 : Selector  InputPortWidth=max(n_actuation,1)  IndexOptions=Index vector (dialog)  Indices=inputselector(2)  OutputSizes=1
  Selector2 : Selector  InputPortWidth=max(n_actuation,1)  IndexOptions=Index vector (dialog)  Indices=inputselector(3)  OutputSizes=1
  Selector3 : Selector  InputPortWidth=max(n_actuation,1)  IndexOptions=Index vector (dialog)  Indices=inputselector(4)  OutputSizes=1
  Selector4 : Selector  InputPortWidth=max(n_actuation,1)  IndexOptions=Index vector (dialog)  Indices=inputselector(5)  OutputSizes=1
  Selector5 : Selector  InputPortWidth=max(n_actuation,1)  IndexOptions=Index vector (dialog)  Indices=inputselector(6)  OutputSizes=1
  A1 : PMIOPort  Port=1  Side=Left
  A6 : PMIOPort  Port=2  Side=Left
  F6 : PMIOPort  Port=3  Side=Left
  F5 : PMIOPort  Port=4  Side=Left
  E5 : PMIOPort  Port=5  Side=Left
  E4 : PMIOPort  Port=6  Side=Left
  B1 : PMIOPort  Port=7  Side=Right
  B2 : PMIOPort  Port=8  Side=Right
  C2 : PMIOPort  Port=9  Side=Right
  C3 : PMIOPort  Port=10  Side=Right
  D3 : PMIOPort  Port=11  Side=Right
  D4 : PMIOPort  Port=12  Side=Right
  Out Bus Element : Outport  PortName=OutBus  Element=Sensing
  wires:
  Foldline5/1 -> Bus Creator4/5
  Selector4/1 -> Foldline5/1
  Drive Function4/1 -> Selector4/1
  Selector3/1 -> Foldline4/1
  Selector2/1 -> Foldline3/1
  Selector1/1 -> Foldline2/1
  Selector/1 -> Foldline1/1
  Drive Function3/1 -> Selector3/1
  Drive Function2/1 -> Selector2/1
  Drive Function1/1 -> Selector1/1
  Foldline2/1 -> Bus Creator4/2
  Foldline3/1 -> Bus Creator4/3
  Foldline4/1 -> Bus Creator4/4
  Foldline1/1 -> Bus Creator4/1
  Drive Function Vector/1 -> Selector/1
  Bus Creator4/1 -> Out Bus Element/1
  Selector5/1 -> Foldline6/1
  Foldline6/1 -> Bus Creator4/6
  Drive Function5/1 -> Selector5/1
  connections:
  Foldline5/RConn1 -- F5/RConn1
  Foldline5/LConn1 -- E5/RConn1
  Foldline2/LConn1 -- C2/RConn1
  Foldline3/RConn1 -- C3/RConn1
  Foldline3/LConn1 -- D3/RConn1
  Foldline4/RConn1 -- E4/RConn1
  Foldline4/LConn1 -- D4/RConn1
  Foldline1/RConn1 -- B1/RConn1
  Foldline1/LConn1 -- A1/RConn1
  Foldline2/RConn1 -- B2/RConn1
  Foldline6/RConn1 -- A6/RConn1
  Foldline6/LConn1 -- F6/RConn1

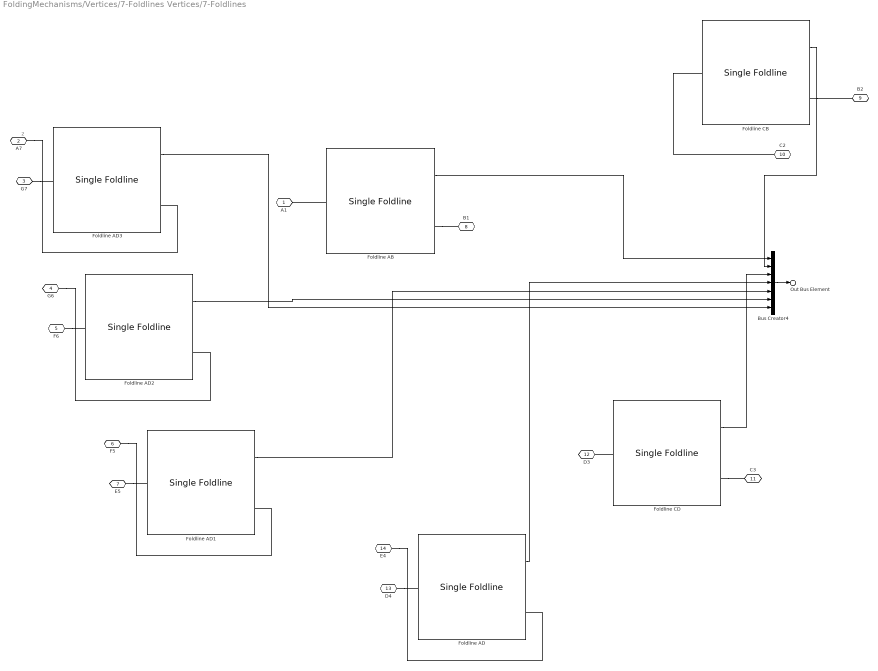
== system FoldingMechanisms/Vertices/7-Foldlines Vertices/7-Foldlines ==
  note: 2
  Bus Creator4 : BusCreator  Inputs=7
  Foldline AB : FoldingMechanisms/Vertices/Subelements/Single Foldline  angleAB=angval(1)  specAngleAB=angspec(1)
      settings: SourceProductName=FoldingMechanisms
  Foldline AD{,1..3} (4 alike) : FoldingMechanisms/Vertices/Subelements/Single Foldline  angleAB=angval(4)  specAngleAB=angspec(4)
      settings: SourceProductName=FoldingMechanisms
  Foldline CB : FoldingMechanisms/Vertices/Subelements/Single Foldline  angleAB=angval(2)  specAngleAB=angspec(2)
      settings: SourceProductName=FoldingMechanisms
  Foldline CD : FoldingMechanisms/Vertices/Subelements/Single Foldline  angleAB=angval(3)  specAngleAB=angspec(2)
      settings: SourceProductName=FoldingMechanisms
  A1 : PMIOPort  Port=1  Side=Left
  A7 : PMIOPort  Port=2  Side=Left
  G7 : PMIOPort  Port=3  Side=Left
  G6 : PMIOPort  Port=4  Side=Left
  F6 : PMIOPort  Port=5  Side=Left
  F5 : PMIOPort  Port=6  Side=Left
  E5 : PMIOPort  Port=7  Side=Left
  B1 : PMIOPort  Port=8  Side=Right
  B2 : PMIOPort  Port=9  Side=Right
  C2 : PMIOPort  Port=10  Side=Right
  C3 : PMIOPort  Port=11  Side=Right
  D3 : PMIOPort  Port=12  Side=Right
  D4 : PMIOPort  Port=13  Side=Right
  E4 : PMIOPort  Port=14  Side=Right
  Out Bus Element : Outport  PortName=OutBus  Element=Sensing
  wires:
  Foldline AD2/1 -> Bus Creator4/6
  Foldline AD1/1 -> Bus Creator4/5
  Foldline CB/1 -> Bus Creator4/2
  Foldline CD/1 -> Bus Creator4/3
  Foldline AD/1 -> Bus Creator4/4
  Foldline AB/1 -> Bus Creator4/1
  Bus Creator4/1 -> Out Bus Element/1
  Foldline AD3/1 -> Bus Creator4/7
  connections:
  G6/RConn1 -- Foldline AD2/RConn1
  F6/RConn1 -- Foldline AD2/LConn1
  E5/RConn1 -- Foldline AD1/LConn1
  F5/RConn1 -- Foldline AD1/RConn1
  C2/RConn1 -- Foldline CB/LConn1
  Foldline CD/RConn1 -- C3/RConn1
  Foldline CD/LConn1 -- D3/RConn1
  E4/RConn1 -- Foldline AD/RConn1
  D4/RConn1 -- Foldline AD/LConn1
  Foldline AB/RConn1 -- B1/RConn1
  Foldline AB/LConn1 -- A1/RConn1
  Foldline CB/RConn1 -- B2/RConn1
  A7/RConn1 -- Foldline AD3/RConn1
  G7/RConn1 -- Foldline AD3/LConn1

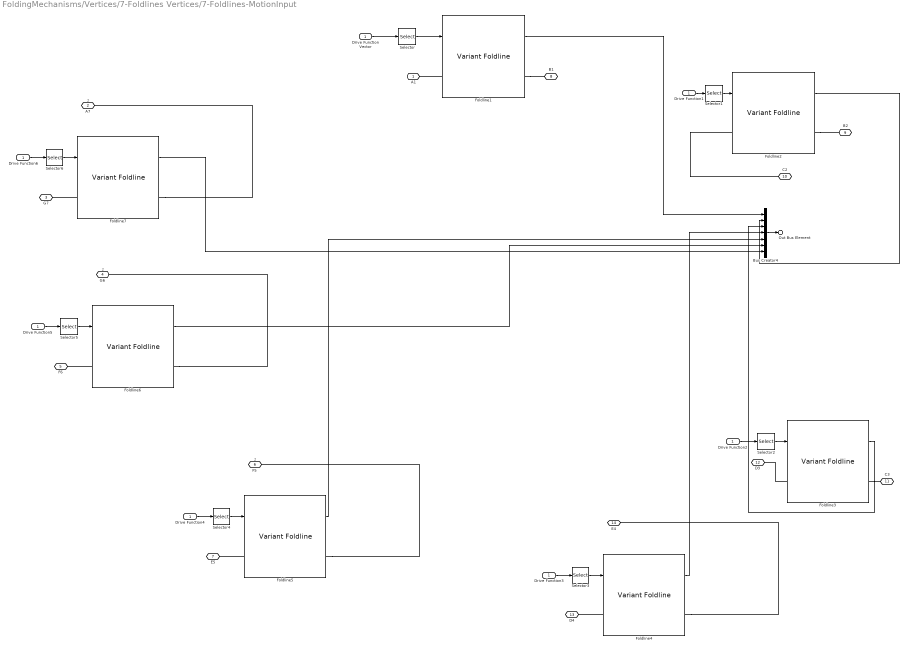
== system FoldingMechanisms/Vertices/7-Foldlines Vertices/7-Foldlines-MotionInput ==
  note: 2
  note: 2
  note: 2
  Drive Function Vector : Inport
  Bus Creator4 : BusCreator  Inputs=7
  Drive Function{1..6} (6 alike) : InportShadow
  Foldline1 : FoldingMechanisms/Vertices/Subelements/Variant Foldline  angleAB=angval(1)  specAngleAB=angspec(1)  actdrive=off  chooseVariant=Foldline
      settings: SourceProductName=FoldingMechanisms
  Foldline2 : FoldingMechanisms/Vertices/Subelements/Variant Foldline  angleAB=angval(2)  specAngleAB=angspec(2)  actdrive=off  chooseVariant=Foldline
      settings: SourceProductName=FoldingMechanisms
  Foldline3 : FoldingMechanisms/Vertices/Subelements/Variant Foldline  angleAB=angval(3)  specAngleAB=angspec(3)  actdrive=off  chooseVariant=Foldline
      settings: SourceProductName=FoldingMechanisms
  Foldline4 : FoldingMechanisms/Vertices/Subelements/Variant Foldline  angleAB=angval(4)  specAngleAB=angspec(4)  actdrive=off  chooseVariant=Foldline
      settings: SourceProductName=FoldingMechanisms
  Foldline5 : FoldingMechanisms/Vertices/Subelements/Variant Foldline  angleAB=angval(5)  specAngleAB=angspec(5)  actdrive=off  chooseVariant=Foldline
      settings: SourceProductName=FoldingMechanisms
  Foldline6 : FoldingMechanisms/Vertices/Subelements/Variant Foldline  angleAB=angval(6)  specAngleAB=angspec(6)  actdrive=off  chooseVariant=Foldline
      settings: SourceProductName=FoldingMechanisms
  Foldline7 : FoldingMechanisms/Vertices/Subelements/Variant Foldline  angleAB=angval(7)  specAngleAB=angspec(7)  actdrive=off  chooseVariant=Foldline
      settings: SourceProductName=FoldingMechanisms
  Selector : Selector  InputPortWidth=max(n_actuation,1)  IndexOptions=Index vector (dialog)  Indices=inputselector(1)  OutputSizes=1
  Selector1 : Selector  InputPortWidth=max(n_actuation,1)  IndexOptions=Index vector (dialog)  Indices=inputselector(2)  OutputSizes=1
  Selector2 : Selector  InputPortWidth=max(n_actuation,1)  IndexOptions=Index vector (dialog)  Indices=inputselector(3)  OutputSizes=1
  Selector3 : Selector  InputPortWidth=max(n_actuation,1)  IndexOptions=Index vector (dialog)  Indices=inputselector(4)  OutputSizes=1
  Selector4 : Selector  InputPortWidth=max(n_actuation,1)  IndexOptions=Index vector (dialog)  Indices=inputselector(5)  OutputSizes=1
  Selector5 : Selector  InputPortWidth=max(n_actuation,1)  IndexOptions=Index vector (dialog)  Indices=inputselector(6)  OutputSizes=1
  Selector6 : Selector  InputPortWidth=max(n_actuation,1)  IndexOptions=Index vector (dialog)  Indices=inputselector(7)  OutputSizes=1
  A1 : PMIOPort  Port=1  Side=Left
  A7 : PMIOPort  Port=2  Side=Left
  G7 : PMIOPort  Port=3  Side=Left
  G6 : PMIOPort  Port=4  Side=Left
  F6 : PMIOPort  Port=5  Side=Left
  F5 : PMIOPort  Port=6  Side=Left
  E5 : PMIOPort  Port=7  Side=Left
  B1 : PMIOPort  Port=8  Side=Right
  B2 : PMIOPort  Port=9  Side=Right
  C2 : PMIOPort  Port=10  Side=Right
  C3 : PMIOPort  Port=11  Side=Right
  D3 : PMIOPort  Port=12  Side=Right
  D4 : PMIOPort  Port=13  Side=Right
  E4 : PMIOPort  Port=14  Side=Right
  Out Bus Element : Outport  PortName=OutBus  Element=Sensing
  wires:
  Foldline5/1 -> Bus Creator4/5
  Selector4/1 -> Foldline5/1
  Drive Function4/1 -> Selector4/1
  Selector3/1 -> Foldline4/1
  Selector2/1 -> Foldline3/1
  Selector1/1 -> Foldline2/1
  Selector/1 -> Foldline1/1
  Drive Function3/1 -> Selector3/1
  Drive Function2/1 -> Selector2/1
  Drive Function1/1 -> Selector1/1
  Foldline2/1 -> Bus Creator4/2
  Foldline3/1 -> Bus Creator4/3
  Foldline4/1 -> Bus Creator4/4
  Foldline1/1 -> Bus Creator4/1
  Drive Function Vector/1 -> Selector/1
  Bus Creator4/1 -> Out Bus Element/1
  Selector5/1 -> Foldline6/1
  Foldline6/1 -> Bus Creator4/6
  Drive Function5/1 -> Selector5/1
  Selector6/1 -> Foldline7/1
  Drive Function6/1 -> Selector6/1
  Foldline7/1 -> Bus Creator4/7
  connections:
  Foldline5/RConn1 -- F5/RConn1
  Foldline5/LConn1 -- E5/RConn1
  Foldline2/LConn1 -- C2/RConn1
  Foldline3/RConn1 -- C3/RConn1
  Foldline3/LConn1 -- D3/RConn1
  Foldline4/RConn1 -- E4/RConn1
  Foldline4/LConn1 -- D4/RConn1
  Foldline1/RConn1 -- B1/RConn1
  Foldline1/LConn1 -- A1/RConn1
  Foldline2/RConn1 -- B2/RConn1
  Foldline6/RConn1 -- G6/RConn1
  Foldline6/LConn1 -- F6/RConn1
  Foldline7/LConn1 -- G7/RConn1
  Foldline7/RConn1 -- A7/RConn1
